simulink model "DiabetesModelProject"  (R2022a)
settings: Solver=VariableStepAuto  StartTime=0.0  StopTime=10  RelTol=1e-3
settings Model: Creator=andy  LastModifiedBy=andy
settings DebuggingCC: UnconnectedInputMsg=warning  UnconnectedOutputMsg=warning  UnconnectedLineMsg=warning
settings RTWCC: DLArmComputeVersion=19.05

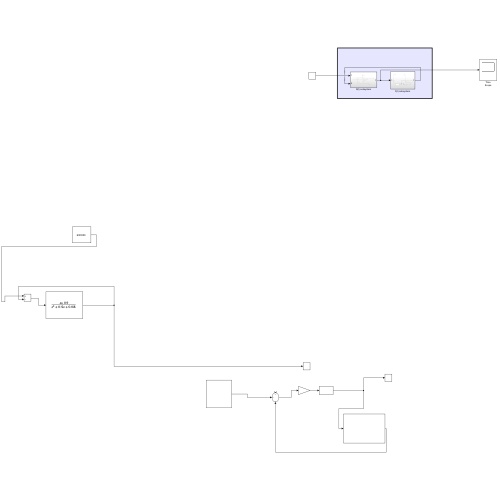
[thumbnail: Simulink's stored preview of the top-level diagram]
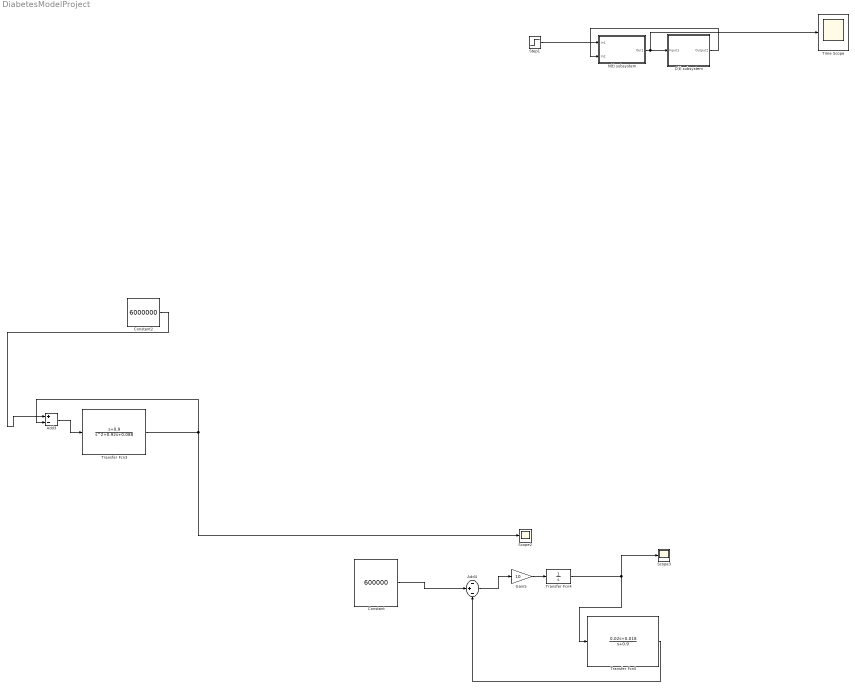
== system DiabetesModelProject ==
  Add3 : Sum  Inputs=+-
  Add4 : Sum  Inputs=-+-
  "C(t) subsystem " : Subsystem
  Constant : Constant  Value=600000
  Constant2 : Constant  Value=6000000
  Gain5 : Gain  Gain=10
  N(t) subsystem : Subsystem
  Scope2 : Scope
  Scope3 : Scope
  Step1 : Step  Time=0  After=6000000  SampleTime=0
  Time Scope : Scope
  Transfer Fcn3 : TransferFcn  Numerator=[1 0.9]  Denominator=[1 0.92 0.088]
  Transfer Fcn4 : TransferFcn  Denominator=[1 0]
  Transfer Fcn5 : TransferFcn  Numerator=[0.02 0.018]  Denominator=[1 0.9]
  wires:
  N(t) subsystem/1(Out1) -> Time Scope/1, "C(t) subsystem "/1(Input1)
  Step1/1 -> N(t) subsystem/1(In1)
  "C(t) subsystem "/1(Output1) -> N(t) subsystem/2(In2)
  Constant2/1 -> Add3/1
  Add3/1 -> Transfer Fcn3/1
  Transfer Fcn3/1 -> Add3/2, Scope2/1
  Add4/1 -> Gain5/1
  Transfer Fcn4/1 -> Scope3/1, Transfer Fcn5/1
  Transfer Fcn5/1 -> Add4/3
  Constant/1 -> Add4/2
  Gain5/1 -> Transfer Fcn4/1

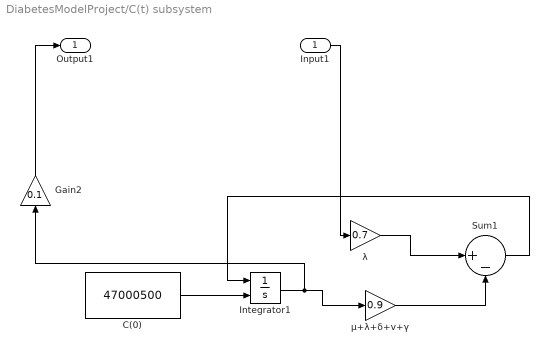
== system DiabetesModelProject/C(t) subsystem  ==
  Input1 : Inport
  C(0) : Constant  Value=47000500
  Gain2 : Gain  Gain=0.1
  Integrator1 : Integrator  InitialConditionSource=external
  Sum1 : Sum  Inputs=|+-
  λ : Gain  Gain=0.7
  μ+λ+δ+v+γ : Gain  Gain=0.9
  Output1 : Outport
  wires:
  λ/1 -> Sum1/1
  Sum1/1 -> Integrator1/1
  Input1/1 -> λ/1
  Integrator1/1 -> μ+λ+δ+v+γ/1, Gain2/1
  Gain2/1 -> Output1/1
  C(0)/1 -> Integrator1/2
  μ+λ+δ+v+γ/1 -> Sum1/2

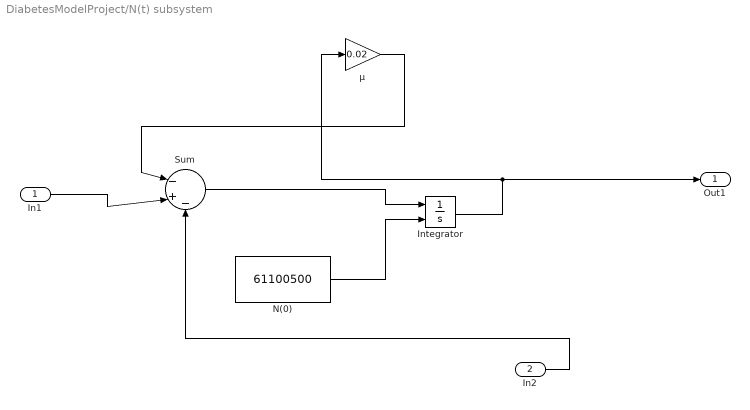
== system DiabetesModelProject/N(t) subsystem ==
  In1 : Inport
  In2 : Inport  Port=2
  Integrator : Integrator  InitialConditionSource=external
  N(0) : Constant  Value=61100500
  Sum : Sum  Inputs=|-+-
  μ : Gain  Gain=0.02
  Out1 : Outport
  wires:
  Sum/1 -> Integrator/1
  N(0)/1 -> Integrator/2
  In2/1 -> Sum/3
  Integrator/1 -> μ/1, Out1/1
  μ/1 -> Sum/1
  In1/1 -> Sum/2
